simulink model "hardware_implementation1"  (R2020a)
settings: Solver=VariableStepAuto  StartTime=0.0  StopTime=10.0  RelTol=1e-3
libraries: arduinolib x6
settings Model: Creator=shobh  LastModifiedBy=shobh

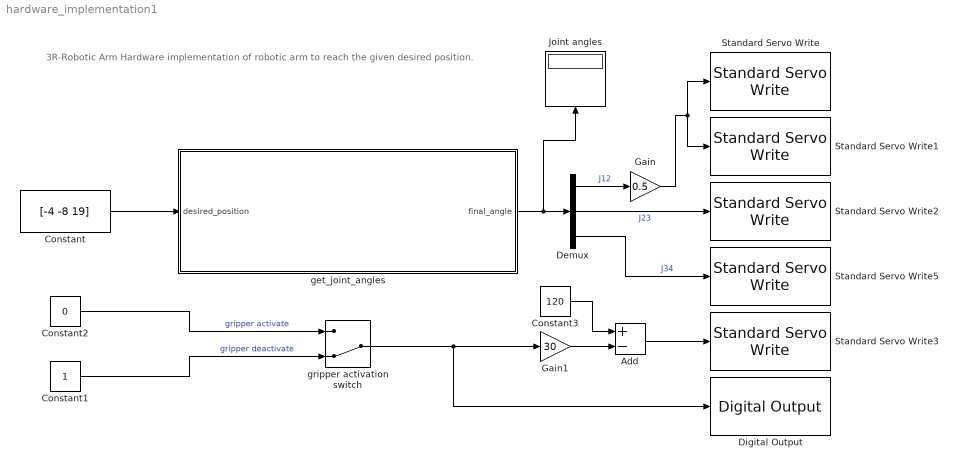
== system hardware_implementation1 ==
  note: 3R-Robotic Arm
      | Hardware implementation of robotic arm to reach the given desired position.
  Add : Sum  Inputs=+-
  Constant : Constant  Value=[-4 -8 19]
  Constant1 : Constant
  Constant2 : Constant  Value=0
  Constant3 : Constant  Value=120
  Demux : Demux  Outputs=3
  Digital Output : arduinolib/Digital Output  pinNumber=11  Direction=output  blockPlatform=arduino
  Gain : Gain  Gain=0.5
  Gain1 : Gain  Gain=30
  Joint angles : Display
  Standard Servo Write : arduinolib/Standard Servo Write  pinNumber=3  ServoIndex=0  blockPlatform=ARDUINO
  Standard Servo Write1 : arduinolib/Standard Servo Write  pinNumber=5  ServoIndex=1  blockPlatform=ARDUINO
  Standard Servo Write2 : arduinolib/Standard Servo Write  pinNumber=6  ServoIndex=2  blockPlatform=ARDUINO
  Standard Servo Write3 : arduinolib/Standard Servo Write  pinNumber=10  ServoIndex=4  blockPlatform=ARDUINO
  Standard Servo Write5 : arduinolib/Standard Servo Write  pinNumber=9  ServoIndex=4  blockPlatform=ARDUINO
  get_joint_angles : Subsystem
  gripper activation switch : ManualSwitch  CurrentSetting=0
  wires:
  Constant1/1 -> gripper activation switch/2  "gripper deactivate"
  Constant2/1 -> gripper activation switch/1  "gripper activate"
  Demux/1 -> Gain/1  "J12"
  Gain/1 -> Standard Servo Write1/1, Standard Servo Write/1
  Constant/1 -> get_joint_angles/1(desired_position)
  Demux/2 -> Standard Servo Write2/1  "J23"
  Demux/3 -> Standard Servo Write5/1  "J34"
  get_joint_angles/1(final_angle) -> Joint angles/1, Demux/1
  Add/1 -> Standard Servo Write3/1
  Constant3/1 -> Add/1
  Gain1/1 -> Add/2
  gripper activation switch/1 -> Gain1/1, Digital Output/1

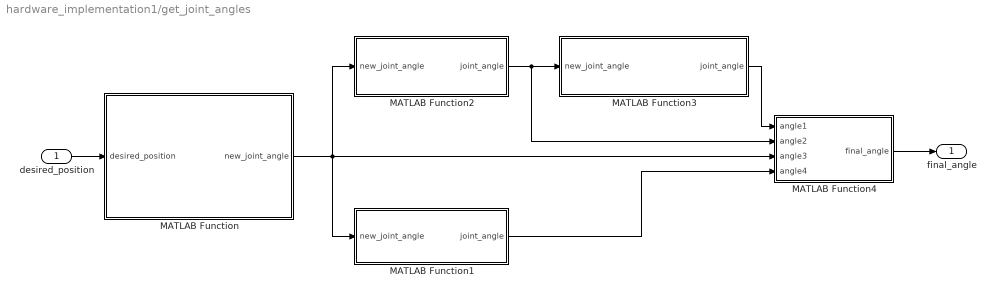
== system hardware_implementation1/get_joint_angles ==
  desired_position : Inport
  MATLAB Function : MATLAB Function  TreatAsAtomicUnit=on
  MATLAB Function1 : MATLAB Function  TreatAsAtomicUnit=on
  MATLAB Function2 : MATLAB Function  TreatAsAtomicUnit=on
  MATLAB Function3 : MATLAB Function  TreatAsAtomicUnit=on
  MATLAB Function4 : MATLAB Function  TreatAsAtomicUnit=on
  final_angle : Outport
  wires:
  desired_position/1 -> MATLAB Function/1(desired_position)
  MATLAB Function/1(new_joint_angle) -> MATLAB Function2/1(new_joint_angle), MATLAB Function4/3(angle3), MATLAB Function1/1(new_joint_angle)
  MATLAB Function2/1(joint_angle) -> MATLAB Function3/1(new_joint_angle), MATLAB Function4/2(angle2)
  MATLAB Function1/1(joint_angle) -> MATLAB Function4/4(angle4)
  MATLAB Function3/1(joint_angle) -> MATLAB Function4/1(angle1)
  MATLAB Function4/1(final_angle) -> final_angle/1

== matlab function hardware_implementation1/get_joint_angles/MATLAB Function ==
  data: desired_position input; new_joint_angle output
function new_joint_angle  = get_angles(desired_position)
    link_length = [10 8 8];
    x = desired_position(1);
    y = desired_position(2);
    z = desired_position(3);
    
    if sqrt(x^2 + y^2) <= link_length(2) + link_length(3)% Check if point is reachable
        q1 = atan2(y, x);
        q3 = acos(((x/cos(q1))^2 + (z-link_length(1))^2 - link_length(2)^2 - link_length(3)^2)/ (2*link_length(2)*link_length(3)));
        q2 = acos(x/(2*link_length(2)*cos(q1)*cos(q3/2))) - (q3/2); % L2 must be equal to L3
        
        if z < link_length(1) % Correcting for angle if point below link_length(1)
            q2 = -q2;
            q3 = -q3;
        end
        
        % Convert angles to range 0 to 2pi
        if q1 < 0 
            q1 = 2*pi + q1;
        end
        if q2 < 0
            q2 = 2*pi + q2;
        end
        if q3 < 0
            q3 = 2*pi + q3;
        end
        
        %If q3 not in range then reset the arm
        if q3 > pi/2 && q3 < 3*pi/2
            new_joint_angle = [0 0 0];
        else
            if mod(floor(q1 * 180/pi), 2) ~=0 % Making the angle q1 even to evenly distribute between two servos 
                q1 = (floor(q1 * 180/pi) - 1)*(pi/180);
            end
            new_joint_angle = floor([q1 q2 q3].*(180/pi));
        end
        
    else
        new_joint_angle = [0 0 0];
    end
end

== matlab function hardware_implementation1/get_joint_angles/MATLAB Function1 ==
  data: new_joint_angle input; joint_angle output
function joint_angle = config4(new_joint_angle)
    
    % Getting the new configuration
    nq3 = 360 - new_joint_angle(3);
    
    nq2 = new_joint_angle(2) - nq3;
    nq3 = -new_joint_angle(3);
   
    % Converting to range [0, 360)
    nq2 = mod(nq2, 360);
    nq3 = mod(nq3, 360);
    
    joint_angle = [new_joint_angle(1) nq2 nq3];
end

== matlab function hardware_implementation1/get_joint_angles/MATLAB Function2 ==
  data: new_joint_angle input; joint_angle output
function joint_angle = config2(new_joint_angle)
    
    % Change the configurations of the angles
    if new_joint_angle(1) >= 0 && new_joint_angle(1) < 180
        q1 = new_joint_angle(1) + 180;
    else
        q1 = new_joint_angle(1) - 180;
    end
    
    q2 = 180 - new_joint_angle(2);
    q3 = -new_joint_angle(3);
    
    % Converting to range [0, 360)
    q2 = mod(q2, 360);
    q3 = mod(q3, 360);
    
    joint_angle = [q1 q2 q3];
end

== matlab function hardware_implementation1/get_joint_angles/MATLAB Function3 ==
  data: new_joint_angle input; joint_angle output
function joint_angle = config3(new_joint_angle)
    
    % Getting the new configuration
    nq3 = 360 - new_joint_angle(3);
    
    nq2 = new_joint_angle(2) - nq3;
    nq3 = -new_joint_angle(3);
    
    % Converting to range [0, 360)
    nq2 = mod(nq2, 360);
    nq3 = mod(nq3, 360);
    
    joint_angle = [new_joint_angle(1) nq2 nq3];
end

== matlab function hardware_implementation1/get_joint_angles/MATLAB Function4 ==
  data: angle1 input; final_angle output; angle2 input; angle3 input; angle4 input
function final_angle = best_config(angle1, angle2, angle3, angle4)
    
    % Check the best joint angle configuration
    if (angle1(2) < 90 || angle1(2) > 270) && (angle1(3) < 90 || angle1(3) > 270)
        final_angle = angle1;
    elseif (angle2(2) < 90 || angle2(2) > 270) && (angle2(3) < 90 || angle2(3) > 270)
        final_angle = angle2;
    elseif (angle3(2) < 90 || angle3(2) > 270) && (angle3(3) < 90 || angle3(3) > 270)
        final_angle = angle3;
    elseif (angle4(2) < 90 || angle4(2) > 270) && (angle4(3) < 90 || angle4(3) > 270)
        final_angle = angle4;
    else
        final_angle = [0 0 0];
    end
    
    % Get servo angle in range of 0 to 180
    if final_angle(2) > 270
        final_angle(2) = final_angle(2) - 270;
    else
        final_angle(2) = 90 + final_angle(2);
    end
    if final_angle(3) > 270
        final_angle(3) = final_angle(3) - 270;
    else
        final_angle(3) = 90 + final_angle(3);
    end
end
